simulink library "Driveline_Axle1_A1Diff"  (R2026a)
settings: Solver=VariableStepAuto
libraries: Driveshaft_Assembly x2, Differential_Systems x1, fl_lib x1, sdl_lib x1
Description:
  | Component of Simscape Vehicle Templates Library
  | 
  | Copyright 2018-2026 The MathWorks, Inc.
settings Model: Creator=smiller  LastModifiedBy=smiller

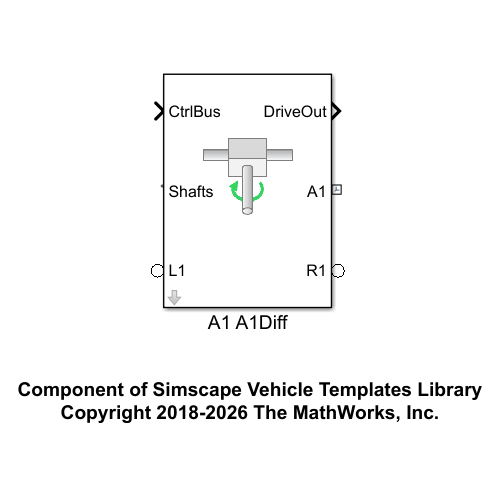
[thumbnail: Simulink's stored preview of the top-level diagram]
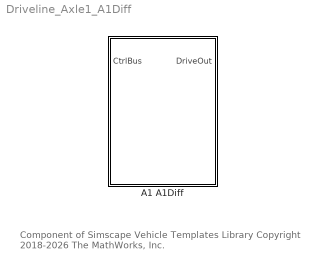
== system Driveline_Axle1_A1Diff ==
  note: Component of Simscape Vehicle Templates Library
      | Copyright 2018-2026 The MathWorks, Inc.
  A1 A1Diff : Subsystem  Tag=PublishSubsystem  VariantControl=IndepFRDiffFDiffR  mask(Driveline, Single-Axle, Single Input Shaft){}
      mask help: Model single-axle driveline with a differential connecting left and right sides.
      mask Display: image('sm_car_vehicle_driveline_axle1_a1_a1diff_IMAGE.png');

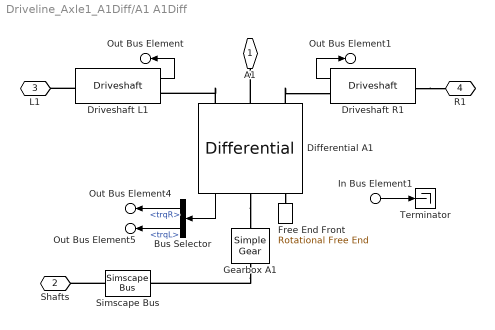
== system Driveline_Axle1_A1Diff/A1 A1Diff ==
  In Bus Element1 : Inport  PortName=CtrlBus
  Bus Selector : BusSelector  OutputSignals=trqR,trqL
  Differential A1 : Differential_Systems/Differential  VariantControl=Variant1  LabelModeActiveChoice=Gear1DShafts1D  Differential=Driveline.DifferentialA1  VariantLabel=Driveline.DifferentialA1.class.Value
      settings: AttributesFormatString=%<ActiveVariant>
  Driveshaft L1 : Driveshaft_Assembly/Driveshaft  VariantControl=Variant1  LabelModeActiveChoice=Shaft1D  popup_leftRight=Left  Driveshaft=Driveline.DriveshaftL1  VariantLabel=Driveline.DriveshaftL1.class.Value
      settings: AttributesFormatString=%<ActiveVariant>
  Driveshaft R1 : Driveshaft_Assembly/Driveshaft  VariantControl=Variant1  LabelModeActiveChoice=Shaft1D  popup_leftRight=Right  Driveshaft=Driveline.DriveshaftR1  VariantLabel=Driveline.DriveshaftR1.class.Value
      settings: AttributesFormatString=%<ActiveVariant>
  Free End Front : fl_lib/Mechanical/Rotational Elements/Rotational Free End  w_specify=off  w_priority=None  w=0 rad/s  w_nominal_specify=off  w_nominal_value=1  w_nominal_unit=rad/s
  Gearbox A1 : sdl_lib/Gears/Simple Gear  ratio=Driveline.GearboxA1.ratio.Value  rotation_direction=3-2*(1)  friction_model=1  T_noload=0.1 N*m  T_nom=5 N*m  efficiency_nom=0.8  efficiency=0.8  temperature_TLU=[280, 300, 320] K  load_TLU=[1, 5, 10] N*m  efficiency_TLU=[.95, .9, .85]  efficiency_TLU2=[.85, .8, .75; .95, .9, .85; .85, .8, .7]  w_thr=0.01 rad/s  pwr_thr=0.001 W  enable_backlash=false  hardstop_model=simscape.enum.hardstop.smooth  backlash_distance=1e-3 mm  r_base=0.1 m  transition=1e-4 mm  backlash_stiffness=1e7 N/m  backlash_damping=1e6 N*s/m  coeff_rest=0  v_tol=0.001 m/s  f_tol=0 N  tau=0.1 s  mu_visc=[0, 0] N*m/(rad/s)  thermal_mass=50 J/K  temperature_specify=off  temperature_priority=High  temperature=300 K  temperature_nominal_specify=off  temperature_nominal_value=1  temperature_nominal_unit=K  x_backlash_specify=off  x_backlash_priority=None  x_backlash=0 mm  x_backlash_nominal_specify=off  x_backlash_nominal_value=1  x_backlash_nominal_unit=mm  f_hardstop_specify=off  f_hardstop_priority=None  f_hardstop=0 N  f_hardstop_nominal_specify=off  f_hardstop_nominal_value=1  f_hardstop_nominal_unit=N  v_backlash_specify=off  v_backlash_priority=None  v_backlash=0 m/s  v_backlash_nominal_specify=off  v_backlash_nominal_value=1  v_backlash_nominal_unit=m/s
  Simscape Bus : SimscapeBus  HierarchyStrings=ShaftA1
  Terminator : Terminator
  A1 : PMIOPort  Side=Right
  Shafts : PMIOPort  Port=2  Side=Left
  L1 : PMIOPort  Port=3  Side=Left
  R1 : PMIOPort  Port=4  Side=Right
  Out Bus Element4 : Outport  VectorParamsAs1DForOutWhenUnconnected=off  PortName=DriveOut  Element=MDriveshaftR1
  Out Bus Element5 : Outport  VectorParamsAs1DForOutWhenUnconnected=off  PortName=DriveOut  Element=MDriveshaftL1
  Out Bus Element : Outport  VectorParamsAs1DForOutWhenUnconnected=off  PortName=DriveOut  Element=anDriveshaftL1
  Out Bus Element1 : Outport  VectorParamsAs1DForOutWhenUnconnected=off  PortName=DriveOut  Element=anDriveshaftR1
  wires:
  Driveshaft R1/1 -> Out Bus Element1/1
  Driveshaft L1/1 -> Out Bus Element/1
  Differential A1/1 -> Bus Selector/1
  Bus Selector/1 -> Out Bus Element4/1  "<trqR>"
  Bus Selector/2 -> Out Bus Element5/1  "<trqL>"
  In Bus Element1/1 -> Terminator/1
  connections:
  Gearbox A1/LConn1 -- Simscape Bus/LConn1
  Differential A1/RConn2 -- Free End Front/LConn1
  Differential A1/LConn1 -- Driveshaft L1/RConn1
  Differential A1/LConn3 -- Driveshaft R1/RConn1
  Driveshaft R1/LConn1 -- R1/RConn1
  Driveshaft L1/LConn1 -- L1/RConn1
  Differential A1/LConn2 -- A1/RConn1
  Differential A1/RConn1 -- Gearbox A1/RConn1
  Simscape Bus/RConn1 -- Shafts/RConn1
